simulink model "ModCin"  (R2023a)
settings: Solver=VariableStepAuto  StartTime=0.0  StopTime=40  RelTol=1e-3
settings Model: Creator=Anita_RR  LastModifiedBy=John_117
settings SolverCC: AlgebraicLoopSolver=TrustRegion
settings DebuggingCC: UnconnectedInputMsg=warning  UnconnectedOutputMsg=warning  UnconnectedLineMsg=warning
settings ModelReferenceCC: EnableRefExpFcnMdlSchedulingChecks=on
settings SFSimCC: CustomCodeUndefinedFunction=UseInterfaceOnly

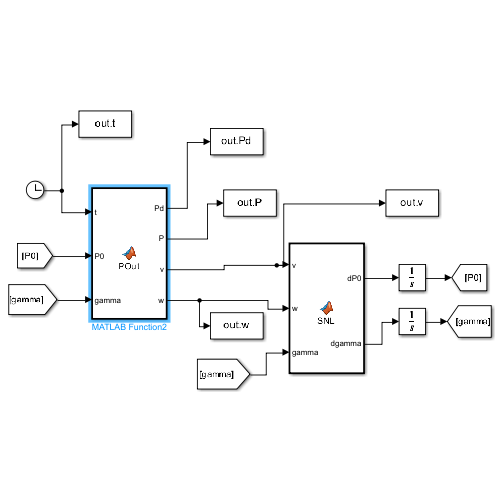
[thumbnail: Simulink's stored preview of the top-level diagram]
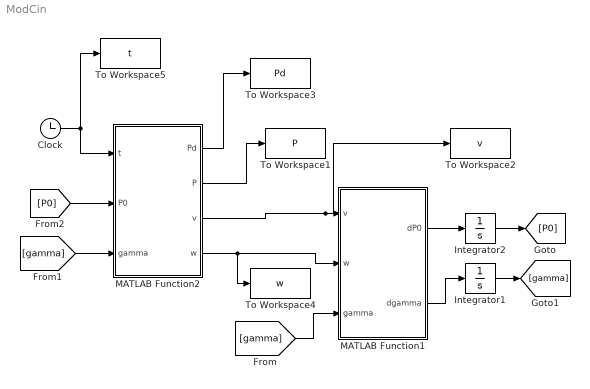
== system ModCin ==
  Clock : Clock
  Integrator1 : Integrator
  Integrator2 : Integrator  InitialCondition=[0;0]
  MATLAB Function1 : MATLAB Function  TreatAsAtomicUnit=on
  MATLAB Function2 : MATLAB Function  TreatAsAtomicUnit=on
  To Workspace1 : ToWorkspace  VariableName=P  SampleTime=-1
      settings: Save2DSignal=2-D array (concatenate along first dimension)
  To Workspace2 : ToWorkspace  VariableName=v  SampleTime=-1
      settings: Save2DSignal=2-D array (concatenate along first dimension)
  To Workspace3 : ToWorkspace  VariableName=Pd  SampleTime=-1
      settings: Save2DSignal=2-D array (concatenate along first dimension)
  To Workspace4 : ToWorkspace  VariableName=w  SampleTime=-1
      settings: Save2DSignal=2-D array (concatenate along first dimension)
  To Workspace5 : ToWorkspace  VariableName=t  SampleTime=-1
      settings: Save2DSignal=2-D array (concatenate along first dimension)
  wires:
  MATLAB Function1/2(dgamma) -> Integrator1/1
  Integrator1/1 -> [gamma]
  Integrator2/1 -> [P0]
  Clock/1 -> To Workspace5/1, MATLAB Function2/1(t)
  [gamma] -> MATLAB Function1/3(gamma)
  MATLAB Function1/1(dP0) -> Integrator2/1
  [P0] -> MATLAB Function2/2(P0)
  [gamma] -> MATLAB Function2/3(gamma)
  MATLAB Function2/1(Pd) -> To Workspace3/1
  MATLAB Function2/2(P) -> To Workspace1/1
  MATLAB Function2/3(v) -> To Workspace2/1, MATLAB Function1/1(v)
  MATLAB Function2/4(w) -> To Workspace4/1, MATLAB Function1/2(w)

== matlab function ModCin/MATLAB Function1 ==
  data: v input; dP0 output; w input; gamma input; dgamma output
function [dP0,dgamma] = SNL(v,w,gamma)
dP0=[v*cos(gamma);v*sin(gamma)];
dgamma=w;

== matlab function ModCin/MATLAB Function2 ==
  data: t input; Pd output; P0 input; gamma input; P output; v output; w output
function [Pd,P,v,w] = POut(t,P0,gamma)
%Control Pd del robot tomando punto por fuera
h=0.1;  kp=2;
%Trayectoria deseada
T=40; b=2*pi/T; %es un circulo
Pd = [cos(b*t); sin(b*t)]; %posicion deseada
dPd = [-b*sin(b*t); b*cos(b*t)]; %derivada de la posicion deseada
%Punto por fuera
P = [P0(1)+h*cos(gamma); P0(2)+h*sin(gamma)]; %coordenadas del punto
%Error del seguimiento
e = Pd-P;
%Matriz de desacoplamiento
A = [cos(gamma), -h*sin(gamma); 
     sin(gamma), h*cos(gamma)];
%Control P con compensacion
u = dPd+kp*e;
U = A\u; %para obtener la matriz inversa de A
v = U(1);
w = U(2);
